simulink model "Microgrid_w_BESS_Q1_1"  (R2024b)
settings: Solver=VariableStepAuto  StartTime=0.0  StopTime=4  RelTol=1e-3
undefined symbols (not defined in the file): ini_SoC, Ion, Lithium, Ts, Ts_Control
libraries: spsParallelRLCBranchLib x8, simulink x6, ee_lib x5, spsSeriesRLCBranchLib x4, nesl_utility x4, spsThreePhaseVIMeasurementLib x3, spsThreePhaseSeriesRLCBranchLib x3, spsCurrentVoltageSimscapeInterfaceLib x3, slpidlib x3, powerlib_extras x3, spsVoltageMeasurementLib x2, spsTwoLevelConverterLib x2
(part 2 of 2)

== matlab function Microgrid_w_BESS_Q1_1/Subsystem/MPPT1/MATLAB Function1 ==
  data: ipv input; Vmpp output; vpv input
function Vmpp = mppt_inccond(ipv, vpv)
    % Incremental Conductance MPPT to output Vmpp
    % Inputs:
    %   ipv - PV current (A)
    %   vpv - PV voltage (V)
    % Output:
    %   Vmpp - Maximum power point voltage (V)

    % Persistent variables to store previous states
    persistent I_prev V_prev Vpv_ref_prev

    % Initialize persistent variables
    if isempty(I_prev)
        I_prev = ipv;
        V_prev = vpv;
        Vpv_ref_prev = 364.5;     % Initial guess near Vmpp
    end

    % Parameters
    delta_Vpv = 1.5;           % Step size for Vpv_ref adjustment
    tol = 1e-4;                % MPP detection tolerance
    v_min = 5;                 % Minimum voltage threshold

    % Handle invalid inputs
    if isnan(ipv) || isnan(vpv) || vpv < v_min
        Vmpp = Vpv_ref_prev;
        return;
    end

    % Incremental Conductance Algorithm
    delta_I = ipv - I_prev;
    delta_V = vpv - V_prev;

    if abs(delta_V) < 1e-4
        if delta_I > 1e-3
            Vpv_ref = Vpv_ref_prev + delta_Vpv;
        elseif delta_I < -1e-3
            Vpv_ref = Vpv_ref_prev - delta_Vpv;
        else
            Vpv_ref = Vpv_ref_prev;
        end
    else
        inst_cond = ipv / vpv;
        inc_cond = delta_I / delta_V;

        if abs(inc_cond + inst_cond) < tol
            Vpv_ref = Vpv_ref_prev;
        elseif inc_cond > -inst_cond
            Vpv_ref = Vpv_ref_prev + delta_Vpv;
        else
            Vpv_ref = Vpv_ref_prev - delta_Vpv;
        end
    end

    % Clamp Vpv_ref to safe range
    Vpv_ref = max(364.5, max(150, Vpv_ref));

    % Output Vmpp
    Vmpp = Vpv_ref;

    % Update states
    I_prev = ipv;
    V_prev = vpv;
    Vpv_ref_prev = Vpv_ref;
end

== matlab function Microgrid_w_BESS_Q1_1/BESS/BATT chg-dshg logic1/MATLAB Function5 ==
  data: Vdc input; D output; Vbatt input; I_batt_meas input; I_batt_ref_mag input; Ts input
function D = controller_discharging(Vdc, Vbatt, I_batt_meas, I_batt_ref_mag, Ts)
%#codegen
% Limits
Imax_discharge = -50;

% PI gains for discharging (tuned for stability and response)
Kp = 0.3; % Increased for faster error correction
Ki = 1; % Moderate integral action with anti-windup
Kd = 0.002; % Derivative term to dampen oscillations
persistent integral_error prev_error prev_I_batt_meas
if isempty(integral_error)
    integral_error = 0;
    prev_error = 0;
    prev_I_batt_meas = 0;
end

% Current reference
I_batt_ref = -I_batt_ref_mag; % Setpoint for discharging (e.g., -20A)

% Clamp current reference
I_batt_ref = max(I_batt_ref, Imax_discharge);

% PI control with derivative and anti-windup
error = I_batt_ref - I_batt_meas;
integral_error = max(min(integral_error + error * Ts, 200), -200); % Anti-windup clamp
derivative = (error - prev_error) / Ts - Kd * (I_batt_meas - prev_I_batt_meas) / Ts; % Damped derivative
PI_output = Kp * error + Ki * integral_error + derivative;
prev_error = error;
prev_I_batt_meas = I_batt_meas;

% Base duty calculation (boost mode)
D_base = 1 - Vbatt / Vdc;

% Total duty with adjusted limits
D = D_base + PI_output;
D = max(min(D, 0.55), 0.127); % New limits: 0.25 to 0.55

% Debugging
assignin('base', 'I_batt_ref', I_batt_ref);
assignin('base', 'I_batt_meas', I_batt_meas);
assignin('base', 'integral_error', integral_error);
assignin('base', 'D', D);
end

== matlab function Microgrid_w_BESS_Q1_1/BESS/BATT chg-dshg logic1/MATLAB Function6 ==
  data: Vdc input; D output; Vbatt input; I_batt_meas input; I_batt_ref_mag input; Ts input
function D = controller_charging(Vdc, Vbatt, I_batt_meas, I_batt_ref_mag, Ts)
%#codegen

% === Controller Parameters ===
Imax_charge = 50;
Kp_i = 2.0;           % Aggressive current loop gain
Ki_i = 20.0;          % Fast integral action
K_d  = 0.01;          % Optional derivative (lead) term

% === Persistent States ===
persistent integral_error_i prev_error_i I_batt_filt
if isempty(integral_error_i)
    integral_error_i = 0;
    prev_error_i = 0;
    I_batt_filt = I_batt_meas;
end

% === Filtered Current Measurement ===
alpha = 0.2;  % Faster response
I_batt_filt = alpha * I_batt_meas + (1 - alpha) * I_batt_filt;

% === Reference Current ===
I_batt_ref = min(I_batt_ref_mag, Imax_charge);  % Clamp ref

% === Skip Voltage Loop for Now ===
I_batt_ref_adj = I_batt_ref;

% === Inner Current Loop ===
error_i = I_batt_ref_adj - I_batt_filt;
d_error_i = (error_i - prev_error_i) / Ts;
prev_error_i = error_i;

PI_output_unsat = Kp_i * error_i + Ki_i * integral_error_i + K_d * d_error_i;

% === Disable Feedforward for Now ===
D_base = 0.5;

% === Saturate Duty and Apply Back-Calculation Anti-Windup ===
D_unsat = D_base + PI_output_unsat;
D_sat = max(min(D_unsat, 0.85), 0.127);
anti_windup_gain = 10;
integral_error_i = integral_error_i + Ts * (error_i + anti_windup_gain * (D_sat - D_unsat));

% === Final Duty Output ===
D = D_sat;

% === Debugging Outputs ===
assignin('base', 'I_batt_ref', I_batt_ref);
assignin('base', 'I_batt_ref_adj', I_batt_ref_adj);
assignin('base', 'I_batt_meas', I_batt_meas);
assignin('base', 'I_batt_filt', I_batt_filt);
assignin('base', 'error_i', error_i);
assignin('base', 'd_error_i', d_error_i);
assignin('base', 'integral_error_i', integral_error_i);
assignin('base', 'PI_output_unsat', PI_output_unsat);
assignin('base', 'D_base', D_base);
assignin('base', 'D_unsat', D_unsat);
assignin('base', 'D', D);
assignin('base', 'Vbatt', Vbatt);
assignin('base', 'Vdc', Vdc);
end

== matlab function Microgrid_w_BESS_Q1_1/Scopes/SoC/MATLAB Function1 ==
  settings: updateMethod=DISCRETE
  data: I_batt input; SoC output; V_batt input; initial_SOC input; Q_nom input; time_scale input; Ts input
function SoC = soc_estimation_with_voltage(I_batt, V_batt, initial_SOC, Q_nom, time_scale, Ts)
%#codegen
% Persistent integrator state
persistent integral_charge SoC_coulomb_state
if isempty(integral_charge)
    integral_charge = 0;
    SoC_coulomb_state = initial_SOC;
end

% Time-scaled charge integration (Ah)
delta_charge = (I_batt * Ts) / 3600; % Positive I_batt means charging
integral_charge = integral_charge + delta_charge * time_scale;

% Update Coulomb-based SoC cumulatively
SoC_coulomb_state = SoC_coulomb_state + (delta_charge * time_scale) / Q_nom;

% Clamp internal state (to prevent runaway)
SoC_coulomb_state = max(0, min(0.9, SoC_coulomb_state));
SoC_coulomb = SoC_coulomb_state;

% Voltage-based correction
V_corr = V_batt - I_batt * 0.1; % R_int = 0.1 Ohm
V_ocv_base = 380 + 50 * SoC_coulomb - 5 * SoC_coulomb^2;
SoC_voltage = max(0, min(1, (V_corr - 380) / 50));  % Linear approximation

% Weighted average
SoC = 0.98 * SoC_coulomb + 0.02 * SoC_voltage;
SoC = max(0, min(0.9, SoC));

% Debugging
assignin('base', 'integral_charge', integral_charge);
assignin('base', 'delta_charge', delta_charge);
assignin('base', 'I_batt', I_batt);
assignin('base', 'SoC_coulomb', SoC_coulomb);
assignin('base', 'SoC_voltage', SoC_voltage);
assignin('base', 'SoC', SoC);
assignin('base', 'V_batt', V_batt);
assignin('base', 'V_ocv_base', V_ocv_base);
assignin('base', 'V_corr', V_corr);
end
